simulink model "case5"  (R2024b)
settings: Solver=FixedStepAuto  StartTime=0  StopTime=1  FixedStep=1e-7  RelTol=1e-3
values from neighbouring files (symbols this model uses):
  SG_D_1_D = 0.01056    [IEEE9_case_parameters.m]    (also in case1_parameters.m; case2_parameters.m; case3_parameters.m; case4_parameters.m)
  SG_D_1_EnableSaturation = 0    [IEEE9_case_parameters.m]    (also in case1_parameters.m; case2_parameters.m; case3_parameters.m; case4_parameters.m)
  SG_D_1_f0 = 60    [IEEE9_case_parameters.m]    (also in case1_parameters.m; case2_parameters.m; case3_parameters.m; case4_parameters.m)
  SG_D_1_H = 7.5    [IEEE9_case_parameters.m]    (also in case1_parameters.m; case2_parameters.m; case3_parameters.m; case4_parameters.m)
  SG_D_1_K_A = 20    [IEEE9_case_parameters.m]    (also in case1_parameters.m; case2_parameters.m; case3_parameters.m; case4_parameters.m)
  SG_D_1_K_E = 1.000000e+1    (= 10)    [IEEE9_case_parameters.m]    (also in case1_parameters.m; case2_parameters.m; case3_parameters.m; case4_parameters.m)
  SG_D_1_K_F = 2.363    [IEEE9_case_parameters.m]    (also in case1_parameters.m; case2_parameters.m; case3_parameters.m; case4_parameters.m)
  SG_D_1_K_s = 0.5    [IEEE9_case_parameters.m]    (also in case1_parameters.m = 5; case2_parameters.m = 5; case3_parameters.m = 5; case4_parameters.m = 5)
  SG_D_1_R_a = 0.001088    [IEEE9_case_parameters.m]    (also in case1_parameters.m; case2_parameters.m; case3_parameters.m; case4_parameters.m)
  SG_D_1_S_A = 1    [IEEE9_case_parameters.m]    (also in case1_parameters.m; case2_parameters.m; case3_parameters.m; case4_parameters.m)
  SG_D_1_S_B = 0.103    [IEEE9_case_parameters.m]    (also in case1_parameters.m; case2_parameters.m; case3_parameters.m; case4_parameters.m)
  SG_D_1_S_N = 10.659857    [IEEE9_case_parameters.m]    (also in case1_parameters.m; case2_parameters.m; case3_parameters.m; case4_parameters.m)
  SG_D_1_SpeedPara = 200    [IEEE9_case_parameters.m]    (also in case1_parameters.m; case2_parameters.m; case3_parameters.m; case4_parameters.m)
  SG_D_1_T_0 = 0.720173    [IEEE9_case_parameters.m]    (also in case1_parameters.m = 0.755522; case2_parameters.m = 0.808931; case3_parameters.m = 0.869402; case4_parameters.m = 0.729316)
  SG_D_1_T_1 = 0.3    [IEEE9_case_parameters.m]    (also in case1_parameters.m; case2_parameters.m; case3_parameters.m; case4_parameters.m)
  SG_D_1_T_2 = 0.05    [IEEE9_case_parameters.m]    (also in case1_parameters.m; case2_parameters.m; case3_parameters.m; case4_parameters.m)
  SG_D_1_T_3 = 0.02    [IEEE9_case_parameters.m]    (also in case1_parameters.m; case2_parameters.m; case3_parameters.m; case4_parameters.m)
  SG_D_1_T_4 = 0.005    [IEEE9_case_parameters.m]    (also in case1_parameters.m; case2_parameters.m; case3_parameters.m; case4_parameters.m)
  SG_D_1_T_A = 0.02    [IEEE9_case_parameters.m]    (also in case1_parameters.m; case2_parameters.m; case3_parameters.m; case4_parameters.m)
  SG_D_1_T_dd = 8.000000e+0    (= 8)    [IEEE9_case_parameters.m]    (also in case1_parameters.m; case2_parameters.m; case3_parameters.m; case4_parameters.m)
  SG_D_1_T_ddd = 0.04    [IEEE9_case_parameters.m]    (also in case1_parameters.m; case2_parameters.m; case3_parameters.m; case4_parameters.m)
  SG_D_1_T_E = 0.314    [IEEE9_case_parameters.m]    (also in case1_parameters.m; case2_parameters.m; case3_parameters.m; case4_parameters.m)
  SG_D_1_T_F = 0.35    [IEEE9_case_parameters.m]    (also in case1_parameters.m; case2_parameters.m; case3_parameters.m; case4_parameters.m)
  SG_D_1_T_qd = 0.8    [IEEE9_case_parameters.m]    (also in case1_parameters.m; case2_parameters.m; case3_parameters.m; case4_parameters.m)
  SG_D_1_T_qdd = 0.02    [IEEE9_case_parameters.m]    (also in case1_parameters.m; case2_parameters.m; case3_parameters.m; case4_parameters.m)
  SG_D_1_T_speed = 0.1    [IEEE9_case_parameters.m]    (also in case1_parameters.m = 200; case2_parameters.m = 200; case3_parameters.m = 200; case4_parameters.m = 200)
  SG_D_1_T_w = 0.5    [IEEE9_case_parameters.m]    (also in case1_parameters.m; case2_parameters.m; case3_parameters.m; case4_parameters.m)
  SG_D_1_V_ref = 1.990276    [IEEE9_case_parameters.m]    (also in case1_parameters.m = 2.042296; case2_parameters.m = 2.051388; case3_parameters.m = 2.089584; case4_parameters.m = 2.01845)
  SG_D_1_w_ref = 376.991118    [IEEE9_case_parameters.m]    (also in case1_parameters.m; case2_parameters.m; case3_parameters.m; case4_parameters.m)
  SG_D_1_wb = 6.000000e+1    (= 60)    [IEEE9_case_parameters.m]    (also in case1_parameters.m; case2_parameters.m; case3_parameters.m; case4_parameters.m)
  SG_D_1_x_d = 1.9    [IEEE9_case_parameters.m]    (also in case1_parameters.m; case2_parameters.m; case3_parameters.m; case4_parameters.m)
  SG_D_1_x_dd = 0.302    [IEEE9_case_parameters.m]    (also in case1_parameters.m; case2_parameters.m; case3_parameters.m; case4_parameters.m)
  SG_D_1_x_ddd = 0.204    [IEEE9_case_parameters.m]    (also in case1_parameters.m; case2_parameters.m; case3_parameters.m; case4_parameters.m)
  SG_D_1_x_l = 0.05    [IEEE9_case_parameters.m]    (also in case1_parameters.m; case2_parameters.m; case3_parameters.m; case4_parameters.m)
  SG_D_1_x_q = 1.3    [IEEE9_case_parameters.m]    (also in case1_parameters.m; case2_parameters.m; case3_parameters.m; case4_parameters.m)
  SG_D_1_x_qd = 0.5    [IEEE9_case_parameters.m]    (also in case1_parameters.m; case2_parameters.m; case3_parameters.m; case4_parameters.m)
  SG_D_1_x_qdd = 0.3    [IEEE9_case_parameters.m]    (also in case1_parameters.m; case2_parameters.m; case3_parameters.m; case4_parameters.m)
  SG_D_2_D = 0.02    [IEEE9_case_parameters.m]    (also in case1_parameters.m; case2_parameters.m; case3_parameters.m; case4_parameters.m)
  SG_D_2_EnableSaturation = 0    [IEEE9_case_parameters.m]    (also in case1_parameters.m; case2_parameters.m; case3_parameters.m; case4_parameters.m)
  SG_D_2_f0 = 60    [IEEE9_case_parameters.m]    (also in case1_parameters.m; case2_parameters.m; case3_parameters.m; case4_parameters.m)
  SG_D_2_H = 8.000000e+0    (= 8)    [IEEE9_case_parameters.m]    (also in case1_parameters.m; case2_parameters.m; case3_parameters.m; case4_parameters.m)
  SG_D_2_K_A = 20    [IEEE9_case_parameters.m]    (also in case1_parameters.m; case2_parameters.m; case3_parameters.m; case4_parameters.m)
  SG_D_2_K_E = 1.000000e+1    (= 10)    [IEEE9_case_parameters.m]    (also in case1_parameters.m; case2_parameters.m; case3_parameters.m; case4_parameters.m)
  SG_D_2_K_F = 2.363    [IEEE9_case_parameters.m]    (also in case1_parameters.m; case2_parameters.m; case3_parameters.m; case4_parameters.m)
  SG_D_2_K_s = 0.5    [IEEE9_case_parameters.m]    (also in case1_parameters.m = 4; case2_parameters.m = 4; case3_parameters.m = 4; case4_parameters.m = 4)
  SG_D_2_R_a = 0.001088    [IEEE9_case_parameters.m]    (also in case1_parameters.m; case2_parameters.m; case3_parameters.m; case4_parameters.m)
  SG_D_2_S_A = 1    [IEEE9_case_parameters.m]    (also in case1_parameters.m; case2_parameters.m; case3_parameters.m; case4_parameters.m)
  SG_D_2_S_B = 0.103    [IEEE9_case_parameters.m]    (also in case1_parameters.m; case2_parameters.m; case3_parameters.m; case4_parameters.m)
  SG_D_2_S_N = 10.659857    [IEEE9_case_parameters.m]    (also in case1_parameters.m; case2_parameters.m; case3_parameters.m; case4_parameters.m)
  SG_D_2_SpeedPara = 200    [IEEE9_case_parameters.m]    (also in case1_parameters.m; case2_parameters.m; case3_parameters.m; case4_parameters.m)
  SG_D_2_T_0 = 1.632913    [IEEE9_case_parameters.m]    (also in case1_parameters.m = 1.632925; case2_parameters.m = 1.632915; case3_parameters.m = 1.632914; case4_parameters.m = 1.632927)
  SG_D_2_T_1 = 0.2    [IEEE9_case_parameters.m]    (also in case1_parameters.m; case2_parameters.m; case3_parameters.m; case4_parameters.m)
  SG_D_2_T_2 = 0.05    [IEEE9_case_parameters.m]    (also in case1_parameters.m; case2_parameters.m; case3_parameters.m; case4_parameters.m)
  SG_D_2_T_3 = 0.02    [IEEE9_case_parameters.m]    (also in case1_parameters.m; case2_parameters.m; case3_parameters.m; case4_parameters.m)
  SG_D_2_T_4 = 0.005    [IEEE9_case_parameters.m]    (also in case1_parameters.m; case2_parameters.m; case3_parameters.m; case4_parameters.m)
  SG_D_2_T_A = 0.02    [IEEE9_case_parameters.m]    (also in case1_parameters.m; case2_parameters.m; case3_parameters.m; case4_parameters.m)
  SG_D_2_T_dd = 7.9    [IEEE9_case_parameters.m]    (also in case1_parameters.m; case2_parameters.m; case3_parameters.m; case4_parameters.m)
  SG_D_2_T_ddd = 0.04    [IEEE9_case_parameters.m]    (also in case1_parameters.m; case2_parameters.m; case3_parameters.m; case4_parameters.m)
  SG_D_2_T_E = 0.314    [IEEE9_case_parameters.m]    (also in case1_parameters.m; case2_parameters.m; case3_parameters.m; case4_parameters.m)
  SG_D_2_T_F = 0.35    [IEEE9_case_parameters.m]    (also in case1_parameters.m; case2_parameters.m; case3_parameters.m; case4_parameters.m)
  SG_D_2_T_qd = 0.8    [IEEE9_case_parameters.m]    (also in case1_parameters.m; case2_parameters.m; case3_parameters.m; case4_parameters.m)
  SG_D_2_T_qdd = 0.015    [IEEE9_case_parameters.m]    (also in case1_parameters.m; case2_parameters.m; case3_parameters.m; case4_parameters.m)
  SG_D_2_T_speed = 0.1    [IEEE9_case_parameters.m]    (also in case1_parameters.m = 150; case2_parameters.m = 150; case3_parameters.m = 150; case4_parameters.m = 150)
  SG_D_2_T_w = 0.35    [IEEE9_case_parameters.m]    (also in case1_parameters.m; case2_parameters.m; case3_parameters.m; case4_parameters.m)
  SG_D_2_V_ref = 2.58547    [IEEE9_case_parameters.m]    (also in case1_parameters.m = 2.597896; case2_parameters.m = 2.587136; case3_parameters.m = 2.586042; case4_parameters.m = 2.599679)
  SG_D_2_w_ref = 376.991118    [IEEE9_case_parameters.m]    (also in case1_parameters.m; case2_parameters.m; case3_parameters.m; case4_parameters.m)
  SG_D_2_wb = 6.000000e+1    (= 60)    [IEEE9_case_parameters.m]    (also in case1_parameters.m; case2_parameters.m; case3_parameters.m; case4_parameters.m)
  SG_D_2_x_d = 1.8    [IEEE9_case_parameters.m]    (also in case1_parameters.m; case2_parameters.m; case3_parameters.m; case4_parameters.m)
  SG_D_2_x_dd = 0.302    [IEEE9_case_parameters.m]    (also in case1_parameters.m; case2_parameters.m; case3_parameters.m; case4_parameters.m)
  SG_D_2_x_ddd = 0.204    [IEEE9_case_parameters.m]    (also in case1_parameters.m; case2_parameters.m; case3_parameters.m; case4_parameters.m)
  SG_D_2_x_l = 0.05    [IEEE9_case_parameters.m]    (also in case1_parameters.m; case2_parameters.m; case3_parameters.m; case4_parameters.m)
  SG_D_2_x_q = 1.25    [IEEE9_case_parameters.m]    (also in case1_parameters.m; case2_parameters.m; case3_parameters.m; case4_parameters.m)
  SG_D_2_x_qd = 0.5    [IEEE9_case_parameters.m]    (also in case1_parameters.m; case2_parameters.m; case3_parameters.m; case4_parameters.m)
  SG_D_2_x_qdd = 0.3    [IEEE9_case_parameters.m]    (also in case1_parameters.m; case2_parameters.m; case3_parameters.m; case4_parameters.m)
  SG_D_3_D = 0.02    [IEEE9_case_parameters.m]    (also in case1_parameters.m; case2_parameters.m; case3_parameters.m; case4_parameters.m)
  SG_D_3_EnableSaturation = 0    [IEEE9_case_parameters.m]    (also in case1_parameters.m; case2_parameters.m; case3_parameters.m; case4_parameters.m)
  SG_D_3_f0 = 60    [IEEE9_case_parameters.m]    (also in case1_parameters.m; case2_parameters.m; case3_parameters.m; case4_parameters.m)
  SG_D_3_H = 7.7    [IEEE9_case_parameters.m]    (also in case1_parameters.m; case2_parameters.m; case3_parameters.m; case4_parameters.m)
  SG_D_3_K_A = 20    [IEEE9_case_parameters.m]    (also in case1_parameters.m; case2_parameters.m; case3_parameters.m; case4_parameters.m)
  SG_D_3_K_E = 1.000000e+1    (= 10)    [IEEE9_case_parameters.m]    (also in case1_parameters.m; case2_parameters.m; case3_parameters.m; case4_parameters.m)
  SG_D_3_K_F = 2.363    [IEEE9_case_parameters.m]    (also in case1_parameters.m; case2_parameters.m; case3_parameters.m; case4_parameters.m)
  SG_D_3_K_s = 0.2    [IEEE9_case_parameters.m]    (also in case1_parameters.m = 2; case2_parameters.m = 2; case3_parameters.m = 2; case4_parameters.m = 2)
  SG_D_3_R_a = 0.001088    [IEEE9_case_parameters.m]    (also in case1_parameters.m; case2_parameters.m; case3_parameters.m; case4_parameters.m)
  SG_D_3_S_A = 1    [IEEE9_case_parameters.m]    (also in case1_parameters.m; case2_parameters.m; case3_parameters.m; case4_parameters.m)
  SG_D_3_S_B = 0.103    [IEEE9_case_parameters.m]    (also in case1_parameters.m; case2_parameters.m; case3_parameters.m; case4_parameters.m)
  SG_D_3_S_N = 10.659857    [IEEE9_case_parameters.m]    (also in case1_parameters.m; case2_parameters.m; case3_parameters.m; case4_parameters.m)
  SG_D_3_SpeedPara = 200    [IEEE9_case_parameters.m]    (also in case1_parameters.m; case2_parameters.m; case3_parameters.m; case4_parameters.m)
  SG_D_3_T_0 = 0.850788    [IEEE9_case_parameters.m]    (also in case1_parameters.m = 0.850786; case2_parameters.m = 0.850787; case3_parameters.m; case4_parameters.m = 0.850786)
  SG_D_3_T_1 = 0.2    [IEEE9_case_parameters.m]    (also in case1_parameters.m; case2_parameters.m; case3_parameters.m; case4_parameters.m)
  SG_D_3_T_2 = 0.05    [IEEE9_case_parameters.m]    (also in case1_parameters.m; case2_parameters.m; case3_parameters.m; case4_parameters.m)
  SG_D_3_T_3 = 0.02    [IEEE9_case_parameters.m]    (also in case1_parameters.m; case2_parameters.m; case3_parameters.m; case4_parameters.m)
  SG_D_3_T_4 = 0.005    [IEEE9_case_parameters.m]    (also in case1_parameters.m; case2_parameters.m; case3_parameters.m; case4_parameters.m)
  SG_D_3_T_A = 0.02    [IEEE9_case_parameters.m]    (also in case1_parameters.m; case2_parameters.m; case3_parameters.m; case4_parameters.m)
  SG_D_3_T_dd = 8.1    [IEEE9_case_parameters.m]    (also in case1_parameters.m; case2_parameters.m; case3_parameters.m; case4_parameters.m)
  SG_D_3_T_ddd = 0.04    [IEEE9_case_parameters.m]    (also in case1_parameters.m; case2_parameters.m; case3_parameters.m; case4_parameters.m)
  SG_D_3_T_E = 0.314    [IEEE9_case_parameters.m]    (also in case1_parameters.m; case2_parameters.m; case3_parameters.m; case4_parameters.m)
  SG_D_3_T_F = 0.35    [IEEE9_case_parameters.m]    (also in case1_parameters.m; case2_parameters.m; case3_parameters.m; case4_parameters.m)
  SG_D_3_T_qd = 0.8    [IEEE9_case_parameters.m]    (also in case1_parameters.m; case2_parameters.m; case3_parameters.m; case4_parameters.m)
  SG_D_3_T_qdd = 0.015    [IEEE9_case_parameters.m]    (also in case1_parameters.m; case2_parameters.m; case3_parameters.m; case4_parameters.m)
  SG_D_3_T_speed = 0.1    [IEEE9_case_parameters.m]    (also in case1_parameters.m = 180; case2_parameters.m = 180; case3_parameters.m = 180; case4_parameters.m = 180)
  SG_D_3_T_w = 0.4    [IEEE9_case_parameters.m]    (also in case1_parameters.m; case2_parameters.m; case3_parameters.m; case4_parameters.m)
  SG_D_3_V_ref = 1.892727    [IEEE9_case_parameters.m]    (also in case1_parameters.m = 1.906439; case2_parameters.m = 1.895535; case3_parameters.m = 1.892105; case4_parameters.m = 1.906598)
  SG_D_3_w_ref = 376.991118    [IEEE9_case_parameters.m]    (also in case1_parameters.m; case2_parameters.m; case3_parameters.m; case4_parameters.m)
  SG_D_3_wb = 6.000000e+1    (= 60)    [IEEE9_case_parameters.m]    (also in case1_parameters.m; case2_parameters.m; case3_parameters.m; case4_parameters.m)
  SG_D_3_x_d = 1.85    [IEEE9_case_parameters.m]    (also in case1_parameters.m; case2_parameters.m; case3_parameters.m; case4_parameters.m)
  SG_D_3_x_dd = 0.302    [IEEE9_case_parameters.m]    (also in case1_parameters.m; case2_parameters.m; case3_parameters.m; case4_parameters.m)
  SG_D_3_x_ddd = 0.204    [IEEE9_case_parameters.m]    (also in case1_parameters.m; case2_parameters.m; case3_parameters.m; case4_parameters.m)
  SG_D_3_x_l = 0.05    [IEEE9_case_parameters.m]    (also in case1_parameters.m; case2_parameters.m; case3_parameters.m; case4_parameters.m)
  SG_D_3_x_q = 1.2    [IEEE9_case_parameters.m]    (also in case1_parameters.m; case2_parameters.m; case3_parameters.m; case4_parameters.m)
  SG_D_3_x_qd = 0.5    [IEEE9_case_parameters.m]    (also in case1_parameters.m; case2_parameters.m; case3_parameters.m; case4_parameters.m)
  SG_D_3_x_qdd = 0.3    [IEEE9_case_parameters.m]    (also in case1_parameters.m; case2_parameters.m; case3_parameters.m; case4_parameters.m)
(part 6 of 12)

== system case5/SG_D_1/d_psi_kq_SG_D_1_block ==
  note: d_psi_kq_SG_D_1 in case5
      | $-\frac{\psi _{\mathrm{gq},\mathrm{SG},D,1}+\psi _{\mathrm{kq},\mathrm{SG},D,1}+\frac{\left(x_{l}-x_{\mathrm{qd}}\right)\,\left(\psi _{q,\mathrm{SG},D,1}+\frac{\psi _{\mathrm{gq},\mathrm{SG},D,1}\,\left(x_{l}-x_{\mathrm{qdd}}\right)}{x_{l}-x_{\mathrm{qd}}}+\frac{\psi _{\mathrm{kq},\mathrm{SG},D,1}\,\left(x_{\mathrm{qd}}-x_{\mathrm{qdd}}\right)}{x_{l}-x_{\mathrm{qd}}}\right)}{x_{\mathrm{qdd}}}}{T_{\mathrm{qdd}}}$
      | Automatically generated on 2025-10-31 19:10:04 .
  State_psi_gq_SG_D_1_d81e0 : Inport
  State_psi_kq_SG_D_1_e8a00 : Inport  Port=2
  State_psi_gq_SG_D_1_5f22b : Inport  Port=3
  State_psi_kq_SG_D_1_7c8e1 : Inport  Port=4
  State_psi_q_SG_D_1_9c6bf : Inport  Port=5
  Add_1b0b3 : Sum
  Add_4cb49 : Sum
  Add_5ccc0 : Sum
  Add_9e13e : Sum
  Add_aefc1 : Sum
  Add_f6ccc : Sum
  Constant_-1_2ccdd : Constant  Value=-1
  Constant_-1_7ac9e : Constant  Value=-1
  Constant_-1_881c4 : Constant  Value=-1
  Constant_-1_8a107 : Constant  Value=-1
  Constant_-1_dc266 : Constant  Value=-1
  Constant_T_qdd_99ceb : Constant  Value=T_qdd
  Constant_x_l_309d0 : Constant  Value=x_l
  Constant_x_l_62d83 : Constant  Value=x_l
  Constant_x_l_b808c : Constant  Value=x_l
  Constant_x_l_c196e : Constant  Value=x_l
  Constant_x_qd_07d99 : Constant  Value=x_qd
  Constant_x_qd_6b8ca : Constant  Value=x_qd
  Constant_x_qd_a0ab1 : Constant  Value=x_qd
  Constant_x_qd_f055d : Constant  Value=x_qd
  Constant_x_qdd_0ca16 : Constant  Value=x_qdd
  Constant_x_qdd_570ed : Constant  Value=x_qdd
  Constant_x_qdd_ad5c1 : Constant  Value=x_qdd
  Divide_06345 : Product  Inputs=*/
  Divide_3d229 : Product  Inputs=*/
  Divide_b3277 : Product  Inputs=*/
  Divide_e408d : Product  Inputs=*/
  Product_1d430 : Product
  Product_1e3da : Product
  Product_5ff23 : Product
  Product_843d3 : Product
  Product_97c23 : Product
  Product_cc1a5 : Product
  Product_dd774 : Product
  Product_e06da : Product
  Subtract_2dff8 : Sum  Inputs=+-
  Subtract_41013 : Sum  Inputs=+-
  Subtract_49882 : Sum  Inputs=+-
  Blockout_d_psi_kq_SG_D_1_2025a : Outport
  wires:
  Product_843d3/1 -> Add_9e13e/1
  Constant_-1_2ccdd/1 -> Product_843d3/1
  Constant_x_l_c196e/1 -> Product_843d3/2
  Constant_x_qdd_0ca16/1 -> Add_9e13e/2
  Constant_-1_dc266/1 -> Product_e06da/1
  Constant_x_qd_f055d/1 -> Subtract_2dff8/1
  Constant_x_qd_6b8ca/1 -> Add_f6ccc/2
  Constant_-1_881c4/1 -> Product_97c23/1
  Constant_x_l_b808c/1 -> Product_e06da/2
  Constant_x_qdd_ad5c1/1 -> Subtract_2dff8/2
  Constant_x_qd_07d99/1 -> Add_4cb49/2
  Constant_x_l_309d0/1 -> Product_97c23/2
  Subtract_49882/1 -> Add_1b0b3/1
  Product_5ff23/1 -> Subtract_49882/1
  State_psi_gq_SG_D_1_5f22b/1 -> Product_cc1a5/1
  Add_9e13e/1 -> Product_cc1a5/2
  Product_97c23/1 -> Add_5ccc0/1
  Constant_x_qd_a0ab1/1 -> Add_5ccc0/2
  State_psi_kq_SG_D_1_7c8e1/1 -> Product_1d430/1
  Product_e06da/1 -> Add_4cb49/1
  Subtract_2dff8/1 -> Product_1d430/2
  Product_cc1a5/1 -> Divide_06345/1
  Add_5ccc0/1 -> Divide_06345/2
  Product_1d430/1 -> Divide_b3277/1
  Add_4cb49/1 -> Divide_b3277/2
  Constant_-1_8a107/1 -> Product_dd774/1
  Constant_x_l_62d83/1 -> Product_dd774/2
  Divide_06345/1 -> Subtract_41013/1
  Divide_b3277/1 -> Subtract_41013/2
  Product_dd774/1 -> Add_f6ccc/1
  Add_aefc1/1 -> Product_1e3da/2
  Subtract_41013/1 -> Add_aefc1/1
  State_psi_q_SG_D_1_9c6bf/1 -> Add_aefc1/2
  Constant_-1_7ac9e/1 -> Product_5ff23/1
  State_psi_gq_SG_D_1_d81e0/1 -> Product_5ff23/2
  Divide_e408d/1 -> Add_1b0b3/2
  Product_1e3da/1 -> Divide_e408d/1
  Add_f6ccc/1 -> Product_1e3da/1
  State_psi_kq_SG_D_1_e8a00/1 -> Subtract_49882/2
  Constant_x_qdd_570ed/1 -> Divide_e408d/2
  Add_1b0b3/1 -> Divide_3d229/1
  Constant_T_qdd_99ceb/1 -> Divide_3d229/2
  Divide_3d229/1 -> Blockout_d_psi_kq_SG_D_1_2025a/1

== system case5/SG_D_1/d_psi_q_SG_D_1_block ==
  note: d_psi_q_SG_D_1 in case5
      | $2\,\pi \,f_{0}\,\left(v_{d,\mathrm{SG},D,1}\,\cos\left(\theta _{\mathrm{SG},D,1}\right)+v_{q,\mathrm{SG},D,1}\,\sin\left(\theta _{\mathrm{SG},D,1}\right)-\frac{R_{a}\,\left(\psi _{q,\mathrm{SG},D,1}+\frac{\psi _{\mathrm{gq},\mathrm{SG},D,1}\,\left(x_{l}-x_{\mathrm{qdd}}\right)}{x_{l}-x_{\mathrm{qd}}}+\frac{\psi _{\mathrm{kq},\mathrm{SG},D,1}\,\left(x_{\mathrm{qd}}-x_{\mathrm{qdd}}\right)}{x_{l}-x_{\mathrm{qd}}}\right)}{x_{\mathrm{qdd}}}-\frac{\psi _{d,\mathrm{SG},D,1}\,w_{\mathrm{SG},D,1}}{2\,f_{0}\,\pi }\right)$
      | Automatically generated on 2025-10-31 19:09:45 .
  State_psi_gq_SG_D_1_86fd1 : Inport
  State_psi_kq_SG_D_1_7a833 : Inport  Port=2
  State_psi_q_SG_D_1_9717c : Inport  Port=3
  Input_v_d_SG_D_1_1af0c : Inport  Port=4
  State_theta_SG_D_1_2d0e9 : Inport  Port=5
  Input_v_q_SG_D_1_f6700 : Inport  Port=6
  State_theta_SG_D_1_d049a : Inport  Port=7
  State_psi_d_SG_D_1_f3a29 : Inport  Port=8
  State_w_SG_D_1_70743 : Inport  Port=9
  Add_0a85e : Sum
  Add_222c1 : Sum
  Add_3e6cd : Sum
  Add_b9156 : Sum
  Add_dad16 : Sum
  Constant_-1_440b8 : Constant  Value=-1
  Constant_-1_6082c : Constant  Value=-1
  Constant_-1_73975 : Constant  Value=-1
  Constant_-2.0_0f128 : Constant  Value=-2.0
  Constant_2.0_f50a3 : Constant  Value=2.0
  Constant_R_a_a467a : Constant  Value=R_a
  Constant_f0_b6ce4 : Constant  Value=f0
  Constant_f0_f1e18 : Constant  Value=f0
  Constant_pi_21fe0 : Constant  Value=pi
  Constant_pi_cf63e : Constant  Value=pi
  Constant_x_l_45d8e : Constant  Value=x_l
  Constant_x_l_95523 : Constant  Value=x_l
  Constant_x_l_ac78d : Constant  Value=x_l
  Constant_x_qd_29703 : Constant  Value=x_qd
  Constant_x_qd_6eda9 : Constant  Value=x_qd
  Constant_x_qd_ed7be : Constant  Value=x_qd
  Constant_x_qdd_6da84 : Constant  Value=x_qdd
  Constant_x_qdd_cd458 : Constant  Value=x_qdd
  Constant_x_qdd_d2184 : Constant  Value=x_qdd
  Divide_2a493 : Product  Inputs=*/
  Divide_2af72 : Product  Inputs=*/
  Divide_6395b : Product  Inputs=*/
  Divide_fcf72 : Product  Inputs=*/
  MathFunc_cos_5a046 : Trigonometry  Operator=cos
  MathFunc_sin_9f6b3 : Trigonometry
  Product_1ef68 : Product
  Product_25b14 : Product
  Product_2bad5 : Product
  Product_3e70f : Product
  Product_4fa79 : Product
  Product_66238 : Product
  Product_69bc1 : Product
  Product_70d97 : Product
  Product_7634e : Product
  Product_7c571 : Product
  Product_aece4 : Product
  Product_b78f3 : Product
  Product_f5fe3 : Product
  Product_fdfb9 : Product
  Subtract_45467 : Sum  Inputs=+-
  Subtract_a2617 : Sum  Inputs=+-
  Subtract_dc1cd : Sum  Inputs=+-
  Subtract_f3c94 : Sum  Inputs=+-
  Blockout_d_psi_q_SG_D_1_385db : Outport
  wires:
  Divide_2a493/1 -> Subtract_a2617/1
  Product_1ef68/1 -> Add_0a85e/1
  Constant_x_l_95523/1 -> Product_1ef68/2
  Constant_-1_73975/1 -> Product_1ef68/1
  Constant_x_qdd_6da84/1 -> Add_0a85e/2
  Constant_x_l_45d8e/1 -> Product_3e70f/2
  Constant_-1_6082c/1 -> Product_3e70f/1
  Constant_x_l_ac78d/1 -> Product_7634e/2
  Constant_x_qdd_d2184/1 -> Subtract_dc1cd/2
  State_psi_kq_SG_D_1_7a833/1 -> Product_2bad5/1
  Constant_-1_440b8/1 -> Product_7634e/1
  Constant_x_qd_6eda9/1 -> Subtract_dc1cd/1
  State_psi_gq_SG_D_1_86fd1/1 -> Product_70d97/1
  Product_7c571/1 -> Blockout_d_psi_q_SG_D_1_385db/1
  Subtract_a2617/1 -> Add_222c1/1
  Product_70d97/1 -> Divide_2a493/1
  Add_0a85e/1 -> Product_70d97/2
  Divide_2af72/1 -> Subtract_a2617/2
  Product_3e70f/1 -> Add_dad16/1
  Constant_x_qd_ed7be/1 -> Add_dad16/2
  Constant_-2.0_0f128/1 -> Product_b78f3/1
  Product_2bad5/1 -> Divide_2af72/1
  Product_7634e/1 -> Add_3e6cd/1
  Subtract_dc1cd/1 -> Product_2bad5/2
  Constant_x_qd_29703/1 -> Add_3e6cd/2
  Add_dad16/1 -> Divide_2a493/2
  Add_3e6cd/1 -> Divide_2af72/2
  Constant_f0_b6ce4/1 -> Product_69bc1/2
  State_psi_q_SG_D_1_9717c/1 -> Add_222c1/2
  Product_4fa79/1 -> Product_fdfb9/1
  Constant_R_a_a467a/1 -> Product_f5fe3/1
  Product_fdfb9/1 -> Divide_fcf72/2
  Product_f5fe3/1 -> Divide_6395b/1
  Add_222c1/1 -> Product_f5fe3/2
  State_theta_SG_D_1_2d0e9/1 -> MathFunc_cos_5a046/1
  Input_v_d_SG_D_1_1af0c/1 -> Product_aece4/1
  Constant_x_qdd_cd458/1 -> Divide_6395b/2
  MathFunc_cos_5a046/1 -> Product_aece4/2
  State_theta_SG_D_1_d049a/1 -> MathFunc_sin_9f6b3/1
  Divide_6395b/1 -> Subtract_45467/1
  Constant_2.0_f50a3/1 -> Product_4fa79/1
  State_w_SG_D_1_70743/1 -> Product_66238/2
  Constant_pi_21fe0/1 -> Product_4fa79/2
  Subtract_f3c94/1 -> Add_b9156/1
  Product_aece4/1 -> Subtract_45467/2
  Divide_fcf72/1 -> Add_b9156/2
  Input_v_q_SG_D_1_f6700/1 -> Product_25b14/1
  MathFunc_sin_9f6b3/1 -> Product_25b14/2
  Product_25b14/1 -> Subtract_f3c94/2
  State_psi_d_SG_D_1_f3a29/1 -> Product_66238/1
  Constant_f0_f1e18/1 -> Product_fdfb9/2
  Constant_pi_cf63e/1 -> Product_b78f3/2
  Subtract_45467/1 -> Subtract_f3c94/1
  Product_66238/1 -> Divide_fcf72/1
  Product_b78f3/1 -> Product_69bc1/1
  Product_69bc1/1 -> Product_7c571/1
  Add_b9156/1 -> Product_7c571/2

== system case5/SG_D_1/d_theta_SG_D_1_block ==
  note: d_theta_SG_D_1 in case5
      | $w_{\mathrm{SG},D,1}-2\,\pi \,f_{0}$
      | Automatically generated on 2025-10-31 19:10:11 .
  State_w_SG_D_1_12e76 : Inport
  Add_34197 : Sum
  Constant_-2.0_e2b98 : Constant  Value=-2.0
  Constant_f0_6e69a : Constant  Value=f0
  Constant_pi_9f9a6 : Constant  Value=pi
  Product_56eaa : Product
  Product_89a4b : Product
  Blockout_d_theta_SG_D_1_084ed : Outport
  wires:
  State_w_SG_D_1_12e76/1 -> Add_34197/2
  Constant_-2.0_e2b98/1 -> Product_89a4b/1
  Constant_f0_6e69a/1 -> Product_56eaa/2
  Constant_pi_9f9a6/1 -> Product_89a4b/2
  Product_56eaa/1 -> Add_34197/1
  Product_89a4b/1 -> Product_56eaa/1
  Add_34197/1 -> Blockout_d_theta_SG_D_1_084ed/1

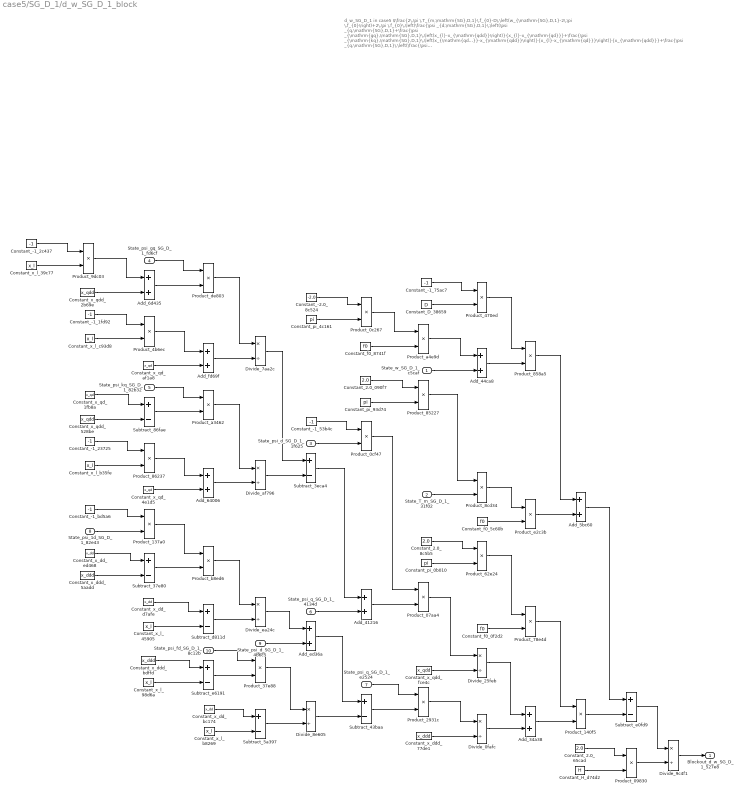
== system case5/SG_D_1/d_w_SG_D_1_block ==
  note: d_w_SG_D_1 in case5
      | $\frac{2\,\pi \,T_{m,\mathrm{SG},D,1}\,f_{0}-D\,\left(w_{\mathrm{SG},D,1}-2\,\pi \,f_{0}\right)+2\,\pi \,f_{0}\,\left(\frac{\psi _{d,\mathrm{SG},D,1}\,\left(\psi _{q,\mathrm{SG},D,1}+\frac{\psi _{\mathrm{gq},\mathrm{SG},D,1}\,\left(x_{l}-x_{\mathrm{qdd}}\right)}{x_{l}-x_{\mathrm{qd}}}+\frac{\psi _{\mathrm{kq},\mathrm{SG},D,1}\,\left(x_{\mathrm{qd}}-x_{\mathrm{qdd}}\right)}{x_{l}-x_{\mathrm{qd}}}\right)}{x_{\mathrm{qdd}}}+\frac{\psi _{q,\mathrm{SG},D,1}\,\left(\frac{\psi _{\mathrm{1d},\mathrm{SG},D,1}\,\left(x_{\mathrm{dd}}-x_{\mathrm{ddd}}\right)}{x_{\mathrm{dd}}-x_{l}}-\psi _{d,\mathrm{SG},D,1}+\frac{\psi _{\mathrm{fd},\mathrm{SG},D,1}\,\left(x_{\mathrm{ddd}}-x_{l}\right)}{x_{\mathrm{dd}}-x_{l}}\right)}{x_{\mathrm{ddd}}}\right)}{2\,H}$
      | Automatically generated on 2025-10-31 19:10:10 .
  State_w_SG_D_1_c5caf : Inport
  State_T_m_SG_D_1_31f02 : Inport  Port=2
  State_psi_d_SG_D_1_1f625 : Inport  Port=3
  State_psi_gq_SG_D_1_fd6cf : Inport  Port=4
  State_psi_kq_SG_D_1_82b32 : Inport  Port=5
  State_psi_q_SG_D_1_4134d : Inport  Port=6
  State_psi_q_SG_D_1_e2524 : Inport  Port=7
  State_psi_1d_SG_D_1_82e43 : Inport  Port=8
  State_psi_d_SG_D_1_4b6c5 : Inport  Port=9
  State_psi_fd_SG_D_1_8c12b : Inport  Port=10
  Add_34a38 : Sum
  Add_41216 : Sum
  Add_44ca8 : Sum
  Add_5bc60 : Sum
  Add_64006 : Sum
  Add_6d435 : Sum
  Add_ed36a : Sum
  Add_fd69f : Sum
  Constant_-1_1fd92 : Constant  Value=-1
  Constant_-1_23725 : Constant  Value=-1
  Constant_-1_2c437 : Constant  Value=-1
  Constant_-1_53b4c : Constant  Value=-1
  Constant_-1_75ac7 : Constant  Value=-1
  Constant_-1_bd5a6 : Constant  Value=-1
  Constant_-2.0_8c524 : Constant  Value=-2.0
  Constant_2.0_090f7 : Constant  Value=2.0
  Constant_2.0_65cad : Constant  Value=2.0
  Constant_2.0_8c5b5 : Constant  Value=2.0
  Constant_D_38659 : Constant  Value=D
  Constant_H_d74d2 : Constant  Value=H
  Constant_f0_0f2d2 : Constant  Value=f0
  Constant_f0_5c60b : Constant  Value=f0
  Constant_f0_8741f : Constant  Value=f0
  Constant_pi_0b010 : Constant  Value=pi
  Constant_pi_4c161 : Constant  Value=pi
  Constant_pi_93d74 : Constant  Value=pi
  Constant_x_dd_bc174 : Constant  Value=x_dd
  Constant_x_dd_d7afe : Constant  Value=x_dd
  Constant_x_dd_ed468 : Constant  Value=x_dd
  Constant_x_ddd_5aadd : Constant  Value=x_ddd
  Constant_x_ddd_77de1 : Constant  Value=x_ddd
  Constant_x_ddd_bdffd : Constant  Value=x_ddd
  Constant_x_l_39c77 : Constant  Value=x_l
  Constant_x_l_45905 : Constant  Value=x_l
  Constant_x_l_98d6a : Constant  Value=x_l
  Constant_x_l_b35fe : Constant  Value=x_l
  Constant_x_l_b8269 : Constant  Value=x_l
  Constant_x_l_c93d8 : Constant  Value=x_l
  Constant_x_qd_1fb8a : Constant  Value=x_qd
  Constant_x_qd_4e1d5 : Constant  Value=x_qd
  Constant_x_qd_af1a8 : Constant  Value=x_qd
  Constant_x_qdd_2b69e : Constant  Value=x_qdd
  Constant_x_qdd_528be : Constant  Value=x_qdd
  Constant_x_qdd_fce4c : Constant  Value=x_qdd
  Divide_0fafc : Product  Inputs=*/
  Divide_25feb : Product  Inputs=*/
  Divide_7aa2c : Product  Inputs=*/
  Divide_8e605 : Product  Inputs=*/
  Divide_9c4f1 : Product  Inputs=*/
  Divide_af796 : Product  Inputs=*/
  Divide_ea24c : Product  Inputs=*/
  Product_07aa4 : Product
  Product_09830 : Product
  Product_0c267 : Product
  Product_0cf47 : Product
  Product_137a0 : Product
  Product_140f5 : Product
  Product_2931c : Product
  Product_37e88 : Product
  Product_470ed : Product
  Product_4b6ec : Product
  Product_62e24 : Product
  Product_78e4d : Product
  Product_85227 : Product
  Product_858a5 : Product
  Product_86237 : Product
  Product_8cd34 : Product
  Product_9dc03 : Product
  Product_a3462 : Product
  Product_a4e9d : Product
  Product_b8ed6 : Product
  Product_de803 : Product
  Product_e2c3b : Product
  Subtract_37e80 : Sum  Inputs=+-
  Subtract_3eca4 : Sum  Inputs=+-
  Subtract_43baa : Sum  Inputs=+-
  Subtract_5a397 : Sum  Inputs=+-
  Subtract_86fae : Sum  Inputs=+-
  Subtract_d811d : Sum  Inputs=+-
  Subtract_e0fd9 : Sum  Inputs=+-
  Subtract_e6191 : Sum  Inputs=+-
  Blockout_d_w_SG_D_1_527e8 : Outport
  wires:
  Product_a4e9d/1 -> Add_44ca8/1
  Constant_-1_2c437/1 -> Product_9dc03/1
  Constant_pi_93d74/1 -> Product_85227/2
  Constant_x_qdd_2b69e/1 -> Add_6d435/2
  Constant_x_l_39c77/1 -> Product_9dc03/2
  Product_9dc03/1 -> Add_6d435/1
  Constant_x_qd_1fb8a/1 -> Subtract_86fae/1
  Constant_-1_1fd92/1 -> Product_4b6ec/1
  Product_0c267/1 -> Product_a4e9d/1
  Constant_x_qdd_528be/1 -> Subtract_86fae/2
  State_psi_q_SG_D_1_e2524/1 -> Product_2931c/1
  Constant_x_l_c93d8/1 -> Product_4b6ec/2
  Constant_-1_23725/1 -> Product_86237/1
  Constant_x_l_b35fe/1 -> Product_86237/2
  Constant_-1_bd5a6/1 -> Product_137a0/1
  Product_4b6ec/1 -> Add_fd69f/1
  State_psi_1d_SG_D_1_82e43/1 -> Product_137a0/2
  Constant_x_dd_ed468/1 -> Subtract_37e80/1
  Subtract_86fae/1 -> Product_a3462/2
  Constant_x_ddd_5aadd/1 -> Subtract_37e80/2
  State_psi_gq_SG_D_1_fd6cf/1 -> Product_de803/1
  Product_0cf47/1 -> Product_07aa4/1
  Add_6d435/1 -> Product_de803/2
  Constant_x_qd_af1a8/1 -> Add_fd69f/2
  State_psi_kq_SG_D_1_82b32/1 -> Product_a3462/1
  Constant_f0_8741f/1 -> Product_a4e9d/2
  Product_86237/1 -> Add_64006/1
  Constant_x_dd_d7afe/1 -> Subtract_d811d/1
  Constant_x_qd_4e1d5/1 -> Add_64006/2
  Product_137a0/1 -> Product_b8ed6/1
  Subtract_37e80/1 -> Product_b8ed6/2
  Constant_x_l_45905/1 -> Subtract_d811d/2
  Constant_x_ddd_bdffd/1 -> Subtract_e6191/1
  Constant_x_l_98d6a/1 -> Subtract_e6191/2
  State_w_SG_D_1_c5caf/1 -> Add_44ca8/2
  Divide_25feb/1 -> Add_34a38/1
  Constant_-1_75ac7/1 -> Product_470ed/1
  Product_de803/1 -> Divide_7aa2c/1
  Add_44ca8/1 -> Product_858a5/2
  Divide_7aa2c/1 -> Subtract_3eca4/1
  Add_fd69f/1 -> Divide_7aa2c/2
  Constant_pi_4c161/1 -> Product_0c267/2
  Product_a3462/1 -> Divide_af796/1
  Add_64006/1 -> Divide_af796/2
  Product_b8ed6/1 -> Divide_ea24c/1
  Divide_ea24c/1 -> Add_ed36a/1
  Subtract_d811d/1 -> Divide_ea24c/2
  State_psi_fd_SG_D_1_8c12b/1 -> Product_37e88/1
  Subtract_e6191/1 -> Product_37e88/2
  Constant_x_dd_bc174/1 -> Subtract_5a397/1
  Constant_x_l_b8269/1 -> Subtract_5a397/2
  Divide_af796/1 -> Subtract_3eca4/2
  Constant_2.0_090f7/1 -> Product_85227/1
  State_psi_d_SG_D_1_4b6c5/1 -> Add_ed36a/2
  Product_37e88/1 -> Divide_8e605/1
  Subtract_5a397/1 -> Divide_8e605/2
  Constant_-2.0_8c524/1 -> Product_0c267/1
  Constant_-1_53b4c/1 -> Product_0cf47/1
  State_psi_d_SG_D_1_1f625/1 -> Product_0cf47/2
  Subtract_3eca4/1 -> Add_41216/1
  Subtract_43baa/1 -> Product_2931c/2
  State_psi_q_SG_D_1_4134d/1 -> Add_41216/2
  Add_ed36a/1 -> Subtract_43baa/1
  Divide_8e605/1 -> Subtract_43baa/2
  Add_41216/1 -> Product_07aa4/2
  Constant_D_38659/1 -> Product_470ed/2
  Product_85227/1 -> Product_8cd34/1
  State_T_m_SG_D_1_31f02/1 -> Product_8cd34/2
  Constant_2.0_8c5b5/1 -> Product_62e24/1
  Constant_pi_0b010/1 -> Product_62e24/2
  Product_07aa4/1 -> Divide_25feb/1
  Constant_x_qdd_fce4c/1 -> Divide_25feb/2
  Product_2931c/1 -> Divide_0fafc/1
  Constant_x_ddd_77de1/1 -> Divide_0fafc/2
  Product_470ed/1 -> Product_858a5/1
  Product_8cd34/1 -> Product_e2c3b/1
  Constant_f0_5c60b/1 -> Product_e2c3b/2
  Product_62e24/1 -> Product_78e4d/1
  Constant_f0_0f2d2/1 -> Product_78e4d/2
  Divide_0fafc/1 -> Add_34a38/2
  Product_858a5/1 -> Add_5bc60/1
  Product_e2c3b/1 -> Add_5bc60/2
  Product_78e4d/1 -> Product_140f5/1
  Add_34a38/1 -> Product_140f5/2
  Add_5bc60/1 -> Subtract_e0fd9/1
  Product_140f5/1 -> Subtract_e0fd9/2
  Constant_2.0_65cad/1 -> Product_09830/1
  Constant_H_d74d2/1 -> Product_09830/2
  Subtract_e0fd9/1 -> Divide_9c4f1/1
  Product_09830/1 -> Divide_9c4f1/2
  Divide_9c4f1/1 -> Blockout_d_w_SG_D_1_527e8/1

== system case5/SG_D_1/i_d_SG_D_1_block ==
  note: i_d_SG_D_1 in case5
      | $\frac{\sin\left(\theta _{\mathrm{SG},D,1}\right)\,\left(\frac{\psi _{\mathrm{1d},\mathrm{SG},D,1}\,\left(x_{\mathrm{dd}}-x_{\mathrm{ddd}}\right)}{x_{\mathrm{dd}}-x_{l}}-\psi _{d,\mathrm{SG},D,1}+\frac{\psi _{\mathrm{fd},\mathrm{SG},D,1}\,\left(x_{\mathrm{ddd}}-x_{l}\right)}{x_{\mathrm{dd}}-x_{l}}\right)}{x_{\mathrm{ddd}}}-\frac{\cos\left(\theta _{\mathrm{SG},D,1}\right)\,\left(\psi _{q,\mathrm{SG},D,1}+\frac{\psi _{\mathrm{gq},\mathrm{SG},D,1}\,\left(x_{l}-x_{\mathrm{qdd}}\right)}{x_{l}-x_{\mathrm{qd}}}+\frac{\psi _{\mathrm{kq},\mathrm{SG},D,1}\,\left(x_{\mathrm{qd}}-x_{\mathrm{qdd}}\right)}{x_{l}-x_{\mathrm{qd}}}\right)}{x_{\mathrm{qdd}}}$
      | Automatically generated on 2025-10-31 19:10:32 .
  State_psi_gq_SG_D_1_bd1f3 : Inport
  State_psi_kq_SG_D_1_c101c : Inport  Port=2
  State_psi_q_SG_D_1_779e3 : Inport  Port=3
  State_theta_SG_D_1_50d30 : Inport  Port=4
  State_psi_1d_SG_D_1_84ef0 : Inport  Port=5
  State_psi_d_SG_D_1_be19d : Inport  Port=6
  State_psi_fd_SG_D_1_58188 : Inport  Port=7
  State_theta_SG_D_1_75ccd : Inport  Port=8
  Add_a0fc6 : Sum
  Add_c32c7 : Sum
  Add_d5621 : Sum
  Add_da1be : Sum
  Add_db6b4 : Sum
  Constant_-1_0c9c0 : Constant  Value=-1
  Constant_-1_39fdf : Constant  Value=-1
  Constant_-1_79eac : Constant  Value=-1
  Constant_-1_8e631 : Constant  Value=-1
  Constant_-1_a1273 : Constant  Value=-1
  Constant_x_dd_105c2 : Constant  Value=x_dd
  Constant_x_dd_31f23 : Constant  Value=x_dd
  Constant_x_dd_d2ccd : Constant  Value=x_dd
  Constant_x_ddd_3d074 : Constant  Value=x_ddd
  Constant_x_ddd_9b1a2 : Constant  Value=x_ddd
  Constant_x_ddd_ff843 : Constant  Value=x_ddd
  Constant_x_l_24f1e : Constant  Value=x_l
  Constant_x_l_4d2aa : Constant  Value=x_l
  Constant_x_l_4ffa6 : Constant  Value=x_l
  Constant_x_l_6fba1 : Constant  Value=x_l
  Constant_x_l_90f73 : Constant  Value=x_l
  Constant_x_l_f0ee4 : Constant  Value=x_l
  Constant_x_qd_0d1e0 : Constant  Value=x_qd
  Constant_x_qd_3c2ec : Constant  Value=x_qd
  Constant_x_qd_70c32 : Constant  Value=x_qd
  Constant_x_qdd_99f1d : Constant  Value=x_qdd
  Constant_x_qdd_a1bc5 : Constant  Value=x_qdd
  Constant_x_qdd_c4452 : Constant  Value=x_qdd
  Divide_7c255 : Product  Inputs=*/
  Divide_c1234 : Product  Inputs=*/
  Divide_cb8bb : Product  Inputs=*/
  Divide_e7253 : Product  Inputs=*/
  Divide_e8747 : Product  Inputs=*/
  Divide_f4ee9 : Product  Inputs=*/
  MathFunc_cos_2bbb8 : Trigonometry  Operator=cos
  MathFunc_sin_464ca : Trigonometry
  Product_07202 : Product
  Product_52ca9 : Product
  Product_9080a : Product
  Product_94da4 : Product
  Product_98370 : Product
  Product_a2715 : Product
  Product_c8d1b : Product
  Product_c9eea : Product
  Product_db878 : Product
  Product_f0d33 : Product
  Product_f5dea : Product
  Subtract_02bda : Sum  Inputs=+-
  Subtract_28b0a : Sum  Inputs=+-
  Subtract_3e06a : Sum  Inputs=+-
  Subtract_60f75 : Sum  Inputs=+-
  Subtract_7686c : Sum  Inputs=+-
  Subtract_81b04 : Sum  Inputs=+-
  Subtract_85f26 : Sum  Inputs=+-
  Subtract_8df87 : Sum  Inputs=+-
  Blockout_i_d_SG_D_1_acf57 : Outport
  wires:
  Constant_-1_79eac/1 -> Product_9080a/1
  Constant_x_l_4d2aa/1 -> Product_9080a/2
  Constant_x_ddd_9b1a2/1 -> Subtract_8df87/2
  Product_9080a/1 -> Add_a0fc6/1
  Constant_x_qdd_c4452/1 -> Subtract_81b04/2
  Constant_x_l_24f1e/1 -> Product_07202/2
  Constant_x_qd_70c32/1 -> Add_c32c7/2
  Constant_x_qdd_99f1d/1 -> Add_a0fc6/2
  Constant_x_qd_3c2ec/1 -> Subtract_81b04/1
  MathFunc_cos_2bbb8/1 -> Product_94da4/2
  Constant_-1_39fdf/1 -> Product_07202/1
  Constant_-1_a1273/1 -> Product_db878/1
  Subtract_85f26/1 -> Blockout_i_d_SG_D_1_acf57/1
  Constant_x_l_4ffa6/1 -> Product_db878/2
  Divide_e8747/1 -> Subtract_7686c/1
  State_psi_gq_SG_D_1_bd1f3/1 -> Product_f0d33/1
  Subtract_60f75/1 -> Product_52ca9/2
  Add_a0fc6/1 -> Product_f0d33/2
  Divide_c1234/1 -> Add_da1be/1
  Product_07202/1 -> Add_d5621/1
  Constant_x_qd_0d1e0/1 -> Add_d5621/2
  State_psi_kq_SG_D_1_c101c/1 -> Product_f5dea/1
  Add_da1be/1 -> Subtract_28b0a/1
  Add_d5621/1 -> Divide_e8747/2
  Subtract_81b04/1 -> Product_f5dea/2
  Product_db878/1 -> Add_c32c7/1
  Constant_-1_8e631/1 -> Product_c8d1b/1
  State_psi_1d_SG_D_1_84ef0/1 -> Product_c8d1b/2
  Constant_x_dd_31f23/1 -> Subtract_8df87/1
  Product_f0d33/1 -> Divide_e8747/1
  Product_a2715/1 -> Divide_cb8bb/1
  Subtract_8df87/1 -> Product_c9eea/2
  Product_f5dea/1 -> Divide_7c255/1
  Product_c8d1b/1 -> Product_c9eea/1
  Add_c32c7/1 -> Divide_7c255/2
  Constant_x_dd_105c2/1 -> Subtract_02bda/1
  Subtract_7686c/1 -> Add_db6b4/1
  Constant_x_l_6fba1/1 -> Subtract_02bda/2
  Constant_x_ddd_ff843/1 -> Subtract_60f75/1
  Constant_x_l_90f73/1 -> Subtract_60f75/2
  Divide_cb8bb/1 -> Subtract_85f26/2
  Divide_7c255/1 -> Subtract_7686c/2
  State_theta_SG_D_1_50d30/1 -> MathFunc_cos_2bbb8/1
  Product_c9eea/1 -> Divide_c1234/1
  Subtract_02bda/1 -> Divide_c1234/2
  State_theta_SG_D_1_75ccd/1 -> MathFunc_sin_464ca/1
  State_psi_fd_SG_D_1_58188/1 -> Product_52ca9/1
  Constant_x_dd_d2ccd/1 -> Subtract_3e06a/1
  Constant_x_l_f0ee4/1 -> Subtract_3e06a/2
  State_psi_q_SG_D_1_779e3/1 -> Add_db6b4/2
  State_psi_d_SG_D_1_be19d/1 -> Add_da1be/2
  Constant_x_ddd_3d074/1 -> Divide_cb8bb/2
  MathFunc_sin_464ca/1 -> Product_a2715/2
  Product_52ca9/1 -> Divide_e7253/1
  Constant_-1_0c9c0/1 -> Product_98370/1
  Subtract_3e06a/1 -> Divide_e7253/2
  Add_db6b4/1 -> Product_98370/2
  Divide_e7253/1 -> Subtract_28b0a/2
  Product_98370/1 -> Product_94da4/1
  Subtract_28b0a/1 -> Product_a2715/1
  Constant_x_qdd_a1bc5/1 -> Divide_f4ee9/2
  Product_94da4/1 -> Divide_f4ee9/1
  Divide_f4ee9/1 -> Subtract_85f26/1

== system case5/SG_D_1/i_q_SG_D_1_block ==
  note: i_q_SG_D_1 in case5
      | $-\frac{\sin\left(\theta _{\mathrm{SG},D,1}\right)\,\left(\psi _{q,\mathrm{SG},D,1}+\frac{\psi _{\mathrm{gq},\mathrm{SG},D,1}\,\left(x_{l}-x_{\mathrm{qdd}}\right)}{x_{l}-x_{\mathrm{qd}}}+\frac{\psi _{\mathrm{kq},\mathrm{SG},D,1}\,\left(x_{\mathrm{qd}}-x_{\mathrm{qdd}}\right)}{x_{l}-x_{\mathrm{qd}}}\right)}{x_{\mathrm{qdd}}}-\frac{\cos\left(\theta _{\mathrm{SG},D,1}\right)\,\left(\frac{\psi _{\mathrm{1d},\mathrm{SG},D,1}\,\left(x_{\mathrm{dd}}-x_{\mathrm{ddd}}\right)}{x_{\mathrm{dd}}-x_{l}}-\psi _{d,\mathrm{SG},D,1}+\frac{\psi _{\mathrm{fd},\mathrm{SG},D,1}\,\left(x_{\mathrm{ddd}}-x_{l}\right)}{x_{\mathrm{dd}}-x_{l}}\right)}{x_{\mathrm{ddd}}}$
      | Automatically generated on 2025-10-31 19:10:36 .
  State_psi_gq_SG_D_1_ce74b : Inport
  State_psi_kq_SG_D_1_d3167 : Inport  Port=2
  State_psi_q_SG_D_1_d260e : Inport  Port=3
  State_theta_SG_D_1_527e7 : Inport  Port=4
  State_psi_1d_SG_D_1_f658e : Inport  Port=5
  State_psi_d_SG_D_1_fbe87 : Inport  Port=6
  State_psi_fd_SG_D_1_7f858 : Inport  Port=7
  State_theta_SG_D_1_42a46 : Inport  Port=8
  Add_13336 : Sum
  Add_450b5 : Sum
  Add_bba6a : Sum
  Add_c7f95 : Sum
  Add_eb689 : Sum
  Add_f7b6a : Sum
  Constant_-1_31947 : Constant  Value=-1
  Constant_-1_5d3be : Constant  Value=-1
  Constant_-1_b81dd : Constant  Value=-1
  Constant_-1_cc0c9 : Constant  Value=-1
  Constant_-1_d99f9 : Constant  Value=-1
  Constant_x_dd_1a9ea : Constant  Value=x_dd
  Constant_x_dd_25323 : Constant  Value=x_dd
  Constant_x_dd_bed85 : Constant  Value=x_dd
  Constant_x_ddd_2cd16 : Constant  Value=x_ddd
  Constant_x_ddd_d046c : Constant  Value=x_ddd
  Constant_x_ddd_eaf7a : Constant  Value=x_ddd
  Constant_x_l_02ad4 : Constant  Value=x_l
  Constant_x_l_0734e : Constant  Value=x_l
  Constant_x_l_15ad6 : Constant  Value=x_l
  Constant_x_l_67863 : Constant  Value=x_l
  Constant_x_l_9dbbe : Constant  Value=x_l
  Constant_x_l_a676f : Constant  Value=x_l
  Constant_x_qd_70e09 : Constant  Value=x_qd
  Constant_x_qd_cbd25 : Constant  Value=x_qd
  Constant_x_qd_e35f2 : Constant  Value=x_qd
  Constant_x_qdd_0e08e : Constant  Value=x_qdd
  Constant_x_qdd_4367b : Constant  Value=x_qdd
  Constant_x_qdd_c823a : Constant  Value=x_qdd
  Divide_10dfb : Product  Inputs=*/
  Divide_4613e : Product  Inputs=*/
  Divide_4cb1c : Product  Inputs=*/
  Divide_6aa59 : Product  Inputs=*/
  Divide_73753 : Product  Inputs=*/
  Divide_c1378 : Product  Inputs=*/
  MathFunc_cos_76f2b : Trigonometry  Operator=cos
  MathFunc_sin_bdd91 : Trigonometry
  Product_05bdb : Product
  Product_0dec9 : Product
  Product_1a669 : Product
  Product_34407 : Product
  Product_5325c : Product
  Product_76214 : Product
  Product_8da53 : Product
  Product_a2a94 : Product
  Product_a4eb5 : Product
  Product_b05f1 : Product
  Product_dbeff : Product
  Subtract_0dff9 : Sum  Inputs=+-
  Subtract_28aeb : Sum  Inputs=+-
  Subtract_67aba : Sum  Inputs=+-
  Subtract_8d8fe : Sum  Inputs=+-
  Subtract_b9cce : Sum  Inputs=+-
  Subtract_d2650 : Sum  Inputs=+-
  Subtract_e723b : Sum  Inputs=+-
  Blockout_i_q_SG_D_1_ba4c2 : Outport
  wires:
  State_theta_SG_D_1_42a46/1 -> MathFunc_cos_76f2b/1
  State_psi_fd_SG_D_1_7f858/1 -> Product_1a669/1
  Constant_-1_b81dd/1 -> Product_0dec9/1
  Constant_x_l_0734e/1 -> Product_0dec9/2
  Subtract_67aba/1 -> Product_1a669/2
  Constant_x_l_a676f/1 -> Subtract_8d8fe/2
  Product_0dec9/1 -> Add_c7f95/1
  Constant_x_qdd_4367b/1 -> Add_c7f95/2
  Constant_x_qd_e35f2/1 -> Subtract_0dff9/1
  Constant_x_qdd_0e08e/1 -> Divide_c1378/2
  MathFunc_sin_bdd91/1 -> Product_76214/2
  Constant_-1_d99f9/1 -> Product_05bdb/1
  Constant_x_qdd_c823a/1 -> Subtract_0dff9/2
  Add_13336/1 -> Product_a2a94/2
  Product_5325c/1 -> Divide_10dfb/1
  Constant_x_l_9dbbe/1 -> Product_05bdb/2
  Constant_-1_cc0c9/1 -> Product_dbeff/1
  Constant_x_l_02ad4/1 -> Product_dbeff/2
  State_psi_gq_SG_D_1_ce74b/1 -> Product_5325c/1
  Add_c7f95/1 -> Product_5325c/2
  Divide_6aa59/1 -> Add_450b5/1
  Product_05bdb/1 -> Add_eb689/1
  Divide_c1378/1 -> Add_f7b6a/1
  Constant_x_qd_cbd25/1 -> Add_eb689/2
  State_psi_kq_SG_D_1_d3167/1 -> Product_b05f1/1
  Add_450b5/1 -> Subtract_e723b/1
  Subtract_0dff9/1 -> Product_b05f1/2
  Divide_10dfb/1 -> Subtract_b9cce/1
  Add_eb689/1 -> Divide_10dfb/2
  Product_dbeff/1 -> Add_bba6a/1
  Constant_x_qd_70e09/1 -> Add_bba6a/2
  Constant_-1_5d3be/1 -> Product_34407/1
  MathFunc_cos_76f2b/1 -> Product_8da53/2
  Product_1a669/1 -> Divide_4613e/1
  State_psi_1d_SG_D_1_f658e/1 -> Product_34407/2
  Constant_x_l_67863/1 -> Subtract_d2650/2
  Constant_x_dd_1a9ea/1 -> Subtract_28aeb/1
  Divide_4613e/1 -> Subtract_e723b/2
  Constant_x_ddd_2cd16/1 -> Subtract_28aeb/2
  Product_8da53/1 -> Divide_4cb1c/1
  Product_b05f1/1 -> Divide_73753/1
  Product_34407/1 -> Product_a4eb5/1
  Add_bba6a/1 -> Divide_73753/2
  Subtract_28aeb/1 -> Product_a4eb5/2
  State_psi_d_SG_D_1_fbe87/1 -> Add_450b5/2
  Constant_x_dd_bed85/1 -> Subtract_8d8fe/1
  Constant_x_ddd_eaf7a/1 -> Subtract_67aba/1
  Constant_x_l_15ad6/1 -> Subtract_67aba/2
  Divide_4cb1c/1 -> Add_f7b6a/2
  Divide_73753/1 -> Subtract_b9cce/2
  State_theta_SG_D_1_527e7/1 -> MathFunc_sin_bdd91/1
  Product_a4eb5/1 -> Divide_6aa59/1
  Subtract_8d8fe/1 -> Divide_6aa59/2
  Constant_x_dd_25323/1 -> Subtract_d2650/1
  Subtract_b9cce/1 -> Add_13336/1
  State_psi_q_SG_D_1_d260e/1 -> Add_13336/2
  Subtract_d2650/1 -> Divide_4613e/2
  Subtract_e723b/1 -> Product_8da53/1
  Constant_-1_31947/1 -> Product_a2a94/1
  Product_a2a94/1 -> Product_76214/1
  Product_76214/1 -> Divide_c1378/1
  Constant_x_ddd_d046c/1 -> Divide_4cb1c/2
  Add_f7b6a/1 -> Blockout_i_q_SG_D_1_ba4c2/1

== system case5/SG_D_1/theta_SG_D_1_out_block ==
  note: theta_SG_D_1_out in case5
      | $\theta _{\mathrm{SG},D,1}$
      | Automatically generated on 2025-10-31 19:10:41 .
  State_theta_SG_D_1_cade5 : Inport
  Blockout_theta_SG_D_1_out_6277a : Outport
  wires:
  State_theta_SG_D_1_cade5/1 -> Blockout_theta_SG_D_1_out_6277a/1

== system case5/SG_D_1/w_SG_D_1_out_block ==
  note: w_SG_D_1_out in case5
      | $w_{\mathrm{SG},D,1}$
      | Automatically generated on 2025-10-31 19:10:41 .
  State_w_SG_D_1_ada09 : Inport
  Blockout_w_SG_D_1_out_7bd8a : Outport
  wires:
  State_w_SG_D_1_ada09/1 -> Blockout_w_SG_D_1_out_7bd8a/1
